simulink model "torque_version"  (R2022a)
settings: Solver=ode15s  StartTime=0.0  StopTime=5  MaxStep=1e-2  RelTol=1e-3
values from neighbouring files (symbols this model uses):
  Disturbance_F = -100    [controller_parameters.m]
  Disturbance_S = 100    [controller_parameters.m]
  k_gn = m*g/0.01    (= 41202)    [controller_parameters.m]
  k_gt = m*g/0.01    (= 41202)    [controller_parameters.m]
  Kd = 10    [controller_parameters.m]
  Kd_pitch = 8    [controller_parameters.m]
  Kp = 100    [controller_parameters.m]
  Kp_pitch = 100    [controller_parameters.m]
  m = 42    [controller_parameters.m]    (also in ground_reaction_params.m = 12)
  m_body = m_total/2    (= 20)    [controller_parameters.m]
  m_legs = m_total/2    (= 20)    [controller_parameters.m]
  mu_slide = 0.8    [controller_parameters.m]    (also in ground_reaction_params.m = 0.008)
  mu_stick = 0.9    [controller_parameters.m]    (also in ground_reaction_params.m = 0.009)
  v_gn_max = 0.03    [controller_parameters.m]
  v_gt_max = 0.03    [controller_parameters.m]
  vLimit = 0.01    [controller_parameters.m]    (also in ground_reaction_params.m = 0.001)
undefined symbols (not defined in the file or in its folder): Newton, Raphson, X, Y, Z
libraries: sm_lib x180, nesl_utility x113, simulink x32, simulink_extras x8
(part 3 of 8)

== system torque_version/Disturbance F ==
  Disturbance : Gain  Gain=Disturbance_F
  Step : Step  Time=2  SampleTime=0
  Step1 : Step  Time=2.1  After=-1  SampleTime=0
  Sum : Sum  Inputs=|++
  Disturbance Force [Frontal] : Outport
  wires:
  Step1/1 -> Sum/2
  Step/1 -> Sum/1
  Disturbance/1 -> Disturbance Force [Frontal]/1
  Sum/1 -> Disturbance/1

== system torque_version/Disturbance S ==
  Disturbance : Gain  Gain=Disturbance_S
  Step : Step  Time=2  SampleTime=0
  Step1 : Step  Time=2.1  After=-1  SampleTime=0
  Sum : Sum  Inputs=|++
  Disturbance Force [Sagittal] : Outport
  wires:
  Step1/1 -> Sum/2
  Step/1 -> Sum/1
  Disturbance/1 -> Disturbance Force [Sagittal]/1
  Sum/1 -> Disturbance/1

== system torque_version/Left Ankle Pitch PD Controller ==
  q : Inport
  dq : Inport  Port=2
  q_ref : Inport  Port=3
  dq_ref : Inport  Port=4
  Enable : EnablePort  StatesWhenEnabling=reset
  KD : Gain  Gain=Kd_pitch
  KP : Gain  Gain=Kp_pitch
  Saturation : Saturate  UpperLimit=40  LowerLimit=-40
  Sum : Sum  Inputs=|+-
  Sum1 : Sum  Inputs=+-|
  Sum2 : Sum  Inputs=|++
  Torque : Outport  OutputWhenDisabled=reset  InitialOutput=0
  wires:
  Saturation/1 -> Torque/1
  Sum2/1 -> Saturation/1
  q/1 -> Sum/2
  KP/1 -> Sum2/2
  dq/1 -> Sum1/2
  q_ref/1 -> Sum/1
  Sum1/1 -> KD/1
  dq_ref/1 -> Sum1/1
  Sum/1 -> KP/1
  KD/1 -> Sum2/1

== system torque_version/Left Ankle Roll PD Controller ==
  q : Inport
  dq : Inport  Port=2
  q_ref : Inport  Port=3
  dq_ref : Inport  Port=4
  Enable : EnablePort  StatesWhenEnabling=reset
  KD : Gain  Gain=Kd
  KP : Gain  Gain=Kp
  Saturation : Saturate  UpperLimit=20  LowerLimit=-20
  Sum : Sum  Inputs=|+-
  Sum1 : Sum  Inputs=+-|
  Sum2 : Sum  Inputs=|++
  Torque : Outport  OutputWhenDisabled=reset  InitialOutput=0
  wires:
  q/1 -> Sum/2
  KP/1 -> Sum2/2
  dq/1 -> Sum1/2
  q_ref/1 -> Sum/1
  Sum1/1 -> KD/1
  dq_ref/1 -> Sum1/1
  Sum/1 -> KP/1
  KD/1 -> Sum2/1
  Sum2/1 -> Saturation/1
  Saturation/1 -> Torque/1

== system torque_version/Left Hip Pitch PD Controller ==
  q : Inport
  dq : Inport  Port=2
  q_ref : Inport  Port=3
  dq_ref : Inport  Port=4
  Enable : EnablePort  StatesWhenEnabling=reset
  KD : Gain  Gain=Kd_pitch
  KP : Gain  Gain=Kp_pitch
  Saturation : Saturate  UpperLimit=50  LowerLimit=-50
  Sum : Sum  Inputs=|+-
  Sum1 : Sum  Inputs=+-|
  Sum2 : Sum  Inputs=|++
  Torque : Outport  OutputWhenDisabled=reset  InitialOutput=0
  wires:
  Saturation/1 -> Torque/1
  Sum2/1 -> Saturation/1
  q/1 -> Sum/2
  KP/1 -> Sum2/2
  dq/1 -> Sum1/2
  q_ref/1 -> Sum/1
  Sum1/1 -> KD/1
  dq_ref/1 -> Sum1/1
  Sum/1 -> KP/1
  KD/1 -> Sum2/1

== system torque_version/Left Hip Roll PD Controller ==
  q : Inport
  dq : Inport  Port=2
  q_ref : Inport  Port=3
  dq_ref : Inport  Port=4
  Enable : EnablePort  StatesWhenEnabling=reset
  KD : Gain  Gain=Kd
  KP : Gain  Gain=Kp
  Saturation : Saturate  UpperLimit=20  LowerLimit=-20
  Sum : Sum  Inputs=|+-
  Sum1 : Sum  Inputs=+-|
  Sum2 : Sum  Inputs=|++
  Torque : Outport  OutputWhenDisabled=reset  InitialOutput=0
  wires:
  KD/1 -> Sum2/1
  Sum/1 -> KP/1
  dq_ref/1 -> Sum1/1
  Sum1/1 -> KD/1
  q_ref/1 -> Sum/1
  dq/1 -> Sum1/2
  KP/1 -> Sum2/2
  q/1 -> Sum/2
  Sum2/1 -> Saturation/1
  Saturation/1 -> Torque/1

== system torque_version/Left Knee Pitch PD Controller ==
  q : Inport
  dq : Inport  Port=2
  q_ref : Inport  Port=3
  dq_ref : Inport  Port=4
  Enable : EnablePort  StatesWhenEnabling=reset
  KD : Gain  Gain=Kd_pitch
  KP : Gain  Gain=Kp_pitch
  Saturation : Saturate  UpperLimit=20  LowerLimit=-20
  Sum : Sum  Inputs=|+-
  Sum1 : Sum  Inputs=+-|
  Sum2 : Sum  Inputs=|++
  Torque : Outport  OutputWhenDisabled=reset  InitialOutput=0
  wires:
  KD/1 -> Sum2/1
  Sum/1 -> KP/1
  dq_ref/1 -> Sum1/1
  Sum1/1 -> KD/1
  q_ref/1 -> Sum/1
  dq/1 -> Sum1/2
  KP/1 -> Sum2/2
  q/1 -> Sum/2
  Sum2/1 -> Saturation/1
  Saturation/1 -> Torque/1

== system torque_version/Right Ankle Pitch PD Controller ==
  q : Inport
  dq : Inport  Port=2
  q_ref : Inport  Port=3
  dq_ref : Inport  Port=4
  Enable : EnablePort  StatesWhenEnabling=reset
  KD : Gain  Gain=Kd_pitch
  KP : Gain  Gain=Kp_pitch
  Saturation : Saturate  UpperLimit=40  LowerLimit=-40
  Sum : Sum  Inputs=|+-
  Sum1 : Sum  Inputs=+-|
  Sum2 : Sum  Inputs=|++
  Torque : Outport  OutputWhenDisabled=reset  InitialOutput=0
  wires:
  KD/1 -> Sum2/1
  Sum/1 -> KP/1
  dq_ref/1 -> Sum1/1
  Sum1/1 -> KD/1
  q_ref/1 -> Sum/1
  dq/1 -> Sum1/2
  KP/1 -> Sum2/2
  q/1 -> Sum/2
  Sum2/1 -> Saturation/1
  Saturation/1 -> Torque/1

== system torque_version/Right Ankle Roll PD Controller ==
  q : Inport
  dq : Inport  Port=2
  q_ref : Inport  Port=3
  dq_ref : Inport  Port=4
  Enable : EnablePort  StatesWhenEnabling=reset
  KD : Gain  Gain=Kd
  KP : Gain  Gain=Kp
  Saturation : Saturate  UpperLimit=20  LowerLimit=-20
  Sum : Sum  Inputs=|+-
  Sum1 : Sum  Inputs=+-|
  Sum2 : Sum  Inputs=|++
  Torque : Outport  OutputWhenDisabled=reset  InitialOutput=0
  wires:
  q/1 -> Sum/2
  KP/1 -> Sum2/2
  dq/1 -> Sum1/2
  q_ref/1 -> Sum/1
  Sum1/1 -> KD/1
  dq_ref/1 -> Sum1/1
  Sum/1 -> KP/1
  KD/1 -> Sum2/1
  Sum2/1 -> Saturation/1
  Saturation/1 -> Torque/1

== system torque_version/Right Hip Pitch PD Controller ==
  q : Inport
  dq : Inport  Port=2
  q_ref : Inport  Port=3
  dq_ref : Inport  Port=4
  Enable : EnablePort  StatesWhenEnabling=reset
  KD : Gain  Gain=Kd_pitch
  KP : Gain  Gain=Kp_pitch
  Saturation : Saturate  UpperLimit=50  LowerLimit=-50
  Sum : Sum  Inputs=|+-
  Sum1 : Sum  Inputs=+-|
  Sum2 : Sum  Inputs=|++
  Torque : Outport  OutputWhenDisabled=reset  InitialOutput=0
  wires:
  KD/1 -> Sum2/1
  Sum/1 -> KP/1
  dq_ref/1 -> Sum1/1
  Sum1/1 -> KD/1
  q_ref/1 -> Sum/1
  dq/1 -> Sum1/2
  KP/1 -> Sum2/2
  q/1 -> Sum/2
  Sum2/1 -> Saturation/1
  Saturation/1 -> Torque/1

== system torque_version/Right Hip Roll PD Controller ==
  q : Inport
  dq : Inport  Port=2
  q_ref : Inport  Port=3
  dq_ref : Inport  Port=4
  Enable : EnablePort  StatesWhenEnabling=reset
  KD : Gain  Gain=Kd
  KP : Gain  Gain=Kp
  Saturation : Saturate  UpperLimit=20  LowerLimit=-20
  Sum : Sum  Inputs=|+-
  Sum1 : Sum  Inputs=+-|
  Sum2 : Sum  Inputs=|++
  Torque : Outport  OutputWhenDisabled=reset  InitialOutput=0
  wires:
  q/1 -> Sum/2
  KP/1 -> Sum2/2
  dq/1 -> Sum1/2
  q_ref/1 -> Sum/1
  Sum1/1 -> KD/1
  dq_ref/1 -> Sum1/1
  Sum/1 -> KP/1
  KD/1 -> Sum2/1
  Sum2/1 -> Saturation/1
  Saturation/1 -> Torque/1

== system torque_version/Right Knee Pitch PD Controller ==
  q : Inport
  dq : Inport  Port=2
  q_ref : Inport  Port=3
  dq_ref : Inport  Port=4
  Enable : EnablePort  StatesWhenEnabling=reset
  KD : Gain  Gain=Kd_pitch
  KP : Gain  Gain=Kp_pitch
  Saturation : Saturate  UpperLimit=20  LowerLimit=-20
  Sum : Sum  Inputs=|+-
  Sum1 : Sum  Inputs=+-|
  Sum2 : Sum  Inputs=|++
  Torque : Outport  OutputWhenDisabled=reset  InitialOutput=0
  wires:
  Saturation/1 -> Torque/1
  Sum2/1 -> Saturation/1
  q/1 -> Sum/2
  KP/1 -> Sum2/2
  dq/1 -> Sum1/2
  q_ref/1 -> Sum/1
  Sum1/1 -> KD/1
  dq_ref/1 -> Sum1/1
  Sum/1 -> KP/1
  KD/1 -> Sum2/1

== system torque_version/Bipedal Model with Torque Control/Left Ball C1 ==
  note: 3D Ground Interaction Model
  Ground : Inport
  3D Contact : Subsystem
  Constant1 : Constant  Value=[0 0 1]
  Demux : Demux  Outputs=3
  Demux1 : Demux  Outputs=3
  External Force and Torque : sm_lib/Forces and Torques/External Force and Torque  ForceResolutionFrame=World  EnableForceX=on  EnableForceY=on  EnableForceZ=on  EnableForce=off  TorqueResolutionFrame=AttachedFrame  EnableTorqueX=off  EnableTorqueY=off  EnableTorqueZ=off  EnableTorque=off
  Mux : Mux  Inputs=3
  Mux1 : Mux  Inputs=3
  Mux2 : Mux  Inputs=3
  PS-Simulink Converter : nesl_utility/PS-Simulink Converter  PhysicalDomain=network_engine_domain  SubClassName=ps_output  LeftPortType=input  RightPortType=output  PseudoPeriodic=off  Frequencies=[]  VectorFormat=1-D array  Unit=m  AffineConversion=off
      settings: SourceProductBaseCode=PW,SS
  PS-Simulink Converter1 : nesl_utility/PS-Simulink Converter  PhysicalDomain=network_engine_domain  SubClassName=ps_output  LeftPortType=input  RightPortType=output  PseudoPeriodic=off  Frequencies=[]  VectorFormat=1-D array  Unit=m  AffineConversion=off
      settings: SourceProductBaseCode=PW,SS
  PS-Simulink Converter2 : nesl_utility/PS-Simulink Converter  PhysicalDomain=network_engine_domain  SubClassName=ps_output  LeftPortType=input  RightPortType=output  PseudoPeriodic=off  Frequencies=[]  VectorFormat=1-D array  Unit=m  AffineConversion=off
      settings: SourceProductBaseCode=PW,SS
  PS-Simulink Converter3 : nesl_utility/PS-Simulink Converter  PhysicalDomain=network_engine_domain  SubClassName=ps_output  LeftPortType=input  RightPortType=output  PseudoPeriodic=off  Frequencies=[]  VectorFormat=1-D array  Unit=m/s  AffineConversion=off
      settings: SourceProductBaseCode=PW,SS
  PS-Simulink Converter4 : nesl_utility/PS-Simulink Converter  PhysicalDomain=network_engine_domain  SubClassName=ps_output  LeftPortType=input  RightPortType=output  PseudoPeriodic=off  Frequencies=[]  VectorFormat=1-D array  Unit=m/s  AffineConversion=off
      settings: SourceProductBaseCode=PW,SS
  PS-Simulink Converter5 : nesl_utility/PS-Simulink Converter  PhysicalDomain=network_engine_domain  SubClassName=ps_output  LeftPortType=input  RightPortType=output  PseudoPeriodic=off  Frequencies=[]  VectorFormat=1-D array  Unit=m/s  AffineConversion=off
      settings: SourceProductBaseCode=PW,SS
  Simulink-PS Converter : nesl_utility/Simulink-PS Converter  PhysicalDomain=network_engine_domain  SubClassName=ps_input  LeftPortType=input  RightPortType=output  PseudoPeriodic=off  Frequencies=[]  NoiseDistribution=none  NoiseParameters=[]  Unit=N  AffineConversion=off  FilteringAndDerivatives=provide  SimscapeFilterOrder=1  InputFilterTimeConstant=0.001  UdotUserProvided=0
      settings: SourceProductBaseCode=PW,SS
  Simulink-PS Converter1 : nesl_utility/Simulink-PS Converter  PhysicalDomain=network_engine_domain  SubClassName=ps_input  LeftPortType=input  RightPortType=output  PseudoPeriodic=off  Frequencies=[]  NoiseDistribution=none  NoiseParameters=[]  Unit=N  AffineConversion=off  FilteringAndDerivatives=provide  SimscapeFilterOrder=1  InputFilterTimeConstant=0.001  UdotUserProvided=0
      settings: SourceProductBaseCode=PW,SS
  Simulink-PS Converter2 : nesl_utility/Simulink-PS Converter  PhysicalDomain=network_engine_domain  SubClassName=ps_input  LeftPortType=input  RightPortType=output  PseudoPeriodic=off  Frequencies=[]  NoiseDistribution=none  NoiseParameters=[]  Unit=N  AffineConversion=off  FilteringAndDerivatives=provide  SimscapeFilterOrder=1  InputFilterTimeConstant=0.001  UdotUserProvided=0
      settings: SourceProductBaseCode=PW,SS
  Sum : Sum  Inputs=|+-
  Sum1 : Sum
  Terminator : Terminator
  Transform Sensor : sm_lib/Frames and Transforms/Transform Sensor  MeasurementFrame=World  SenseAngle=off  SenseAxis=off  SenseAngle1=off  SenseAngle2=off  SenseAngle3=off  SenseQ=off  SenseR=off  SenseOmegaX=off  SenseOmegaY=off  SenseOmegaZ=off  SenseOmega1=off  SenseOmega2=off  SenseOmega3=off  SenseQDot=off  SenseRDot=off  SenseAlphaX=off  SenseAlphaY=off  SenseAlphaZ=off  SenseAlpha1=off  SenseAlpha2=off  SenseAlpha3=off  SenseQDDot=off  SenseRDDot=off  SenseX=on  SenseY=on  SenseZ=on  SenseRad=off  SenseAzim=off  SenseDist=off  SenseInc=off  SenseXDot=on  SenseYDot=on  SenseZDot=on  SenseRadDot=off  SenseAzimDot=off  SenseDistDot=off  SenseIncDot=off  SenseXDDot=off  SenseYDDot=off  SenseZDDot=off  SenseRadDDot=off  SenseAzimDDot=off  SenseDistDDot=off  SenseIncDDot=off
  contact? : simulink/Logic and Bit Operations/Compare To Zero  relop=<=  OutDataTypeStr=boolean
  z : Selector  InputPortWidth=3  IndexOptions=Index vector (dialog)  Indices=3  OutputSizes=1
  F : PMIOPort  Side=Left
  WorldFrame : PMIOPort  Port=2  Side=Left
  RBallCnt : Outport
  GRF [N N N] : Outport  Port=2
  GRFt [N N N] : Outport  Port=3
  GRFn [N N N] : Outport  Port=4
  wires:
  contact?/1 -> 3D Contact/Enable, RBallCnt/1  "cnt"
  Mux2/1 -> 3D Contact/4(vVec [m/s m/s m/s])
  3D Contact/1(FnVec [N N N]) -> Sum1/1, GRFn [N N N]/1
  3D Contact/2(FtVec [N N N]) -> Sum1/2, GRFt [N N N]/1
  Sum1/1 -> GRF [N N N]/1, Demux1/1
  Sum/1 -> contact?/1
  z/1 -> Sum/1
  Ground/1 -> Mux/3, Sum/2  "EnvHeight"
  Constant1/1 -> 3D Contact/2(nVec [m m m])  "Normal Vector nVec"
  Mux1/1 -> 3D Contact/3(pVec [m m m]), z/1, Demux/1  "Reference Point RefPt"
  Demux/1 -> Mux/1
  Mux/1 -> 3D Contact/1(RefPt [m m m])
  Demux1/1 -> Simulink-PS Converter/1
  Demux1/2 -> Simulink-PS Converter1/1
  Demux1/3 -> Simulink-PS Converter2/1
  PS-Simulink Converter1/1 -> Mux1/2
  PS-Simulink Converter/1 -> Mux1/1
  PS-Simulink Converter2/1 -> Mux1/3
  PS-Simulink Converter3/1 -> Mux2/1
  PS-Simulink Converter4/1 -> Mux2/2
  PS-Simulink Converter5/1 -> Mux2/3
  Demux/3 -> Terminator/1
  Demux/2 -> Mux/2
  connections:
  Transform Sensor/RConn1 -- External Force and Torque/RConn1 -- F/RConn1
  Simulink-PS Converter/RConn1 -- External Force and Torque/LConn1
  Simulink-PS Converter1/RConn1 -- External Force and Torque/LConn2
  Simulink-PS Converter2/RConn1 -- External Force and Torque/LConn3
  WorldFrame/RConn1 -- Transform Sensor/LConn1
  PS-Simulink Converter/LConn1 -- Transform Sensor/RConn2
  PS-Simulink Converter1/LConn1 -- Transform Sensor/RConn3
  PS-Simulink Converter2/LConn1 -- Transform Sensor/RConn4
  PS-Simulink Converter3/LConn1 -- Transform Sensor/RConn5
  PS-Simulink Converter4/LConn1 -- Transform Sensor/RConn6
  PS-Simulink Converter5/LConn1 -- Transform Sensor/RConn7

== system torque_version/Bipedal Model with Torque Control/Left Ball C2 ==
  note: 3D Ground Interaction Model
  Ground : Inport
  3D Contact : Subsystem
  Constant1 : Constant  Value=[0 0 1]
  Demux : Demux  Outputs=3
  Demux1 : Demux  Outputs=3
  External Force and Torque : sm_lib/Forces and Torques/External Force and Torque  ForceResolutionFrame=World  EnableForceX=on  EnableForceY=on  EnableForceZ=on  EnableForce=off  TorqueResolutionFrame=AttachedFrame  EnableTorqueX=off  EnableTorqueY=off  EnableTorqueZ=off  EnableTorque=off
  Mux : Mux  Inputs=3
  Mux1 : Mux  Inputs=3
  Mux2 : Mux  Inputs=3
  PS-Simulink Converter : nesl_utility/PS-Simulink Converter  PhysicalDomain=network_engine_domain  SubClassName=ps_output  LeftPortType=input  RightPortType=output  PseudoPeriodic=off  Frequencies=[]  VectorFormat=1-D array  Unit=m  AffineConversion=off
      settings: SourceProductBaseCode=PW,SS
  PS-Simulink Converter1 : nesl_utility/PS-Simulink Converter  PhysicalDomain=network_engine_domain  SubClassName=ps_output  LeftPortType=input  RightPortType=output  PseudoPeriodic=off  Frequencies=[]  VectorFormat=1-D array  Unit=m  AffineConversion=off
      settings: SourceProductBaseCode=PW,SS
  PS-Simulink Converter2 : nesl_utility/PS-Simulink Converter  PhysicalDomain=network_engine_domain  SubClassName=ps_output  LeftPortType=input  RightPortType=output  PseudoPeriodic=off  Frequencies=[]  VectorFormat=1-D array  Unit=m  AffineConversion=off
      settings: SourceProductBaseCode=PW,SS
  PS-Simulink Converter3 : nesl_utility/PS-Simulink Converter  PhysicalDomain=network_engine_domain  SubClassName=ps_output  LeftPortType=input  RightPortType=output  PseudoPeriodic=off  Frequencies=[]  VectorFormat=1-D array  Unit=m/s  AffineConversion=off
      settings: SourceProductBaseCode=PW,SS
  PS-Simulink Converter4 : nesl_utility/PS-Simulink Converter  PhysicalDomain=network_engine_domain  SubClassName=ps_output  LeftPortType=input  RightPortType=output  PseudoPeriodic=off  Frequencies=[]  VectorFormat=1-D array  Unit=m/s  AffineConversion=off
      settings: SourceProductBaseCode=PW,SS
  PS-Simulink Converter5 : nesl_utility/PS-Simulink Converter  PhysicalDomain=network_engine_domain  SubClassName=ps_output  LeftPortType=input  RightPortType=output  PseudoPeriodic=off  Frequencies=[]  VectorFormat=1-D array  Unit=m/s  AffineConversion=off
      settings: SourceProductBaseCode=PW,SS
  Simulink-PS Converter : nesl_utility/Simulink-PS Converter  PhysicalDomain=network_engine_domain  SubClassName=ps_input  LeftPortType=input  RightPortType=output  PseudoPeriodic=off  Frequencies=[]  NoiseDistribution=none  NoiseParameters=[]  Unit=N  AffineConversion=off  FilteringAndDerivatives=provide  SimscapeFilterOrder=1  InputFilterTimeConstant=0.001  UdotUserProvided=0
      settings: SourceProductBaseCode=PW,SS
  Simulink-PS Converter1 : nesl_utility/Simulink-PS Converter  PhysicalDomain=network_engine_domain  SubClassName=ps_input  LeftPortType=input  RightPortType=output  PseudoPeriodic=off  Frequencies=[]  NoiseDistribution=none  NoiseParameters=[]  Unit=N  AffineConversion=off  FilteringAndDerivatives=provide  SimscapeFilterOrder=1  InputFilterTimeConstant=0.001  UdotUserProvided=0
      settings: SourceProductBaseCode=PW,SS
  Simulink-PS Converter2 : nesl_utility/Simulink-PS Converter  PhysicalDomain=network_engine_domain  SubClassName=ps_input  LeftPortType=input  RightPortType=output  PseudoPeriodic=off  Frequencies=[]  NoiseDistribution=none  NoiseParameters=[]  Unit=N  AffineConversion=off  FilteringAndDerivatives=provide  SimscapeFilterOrder=1  InputFilterTimeConstant=0.001  UdotUserProvided=0
      settings: SourceProductBaseCode=PW,SS
  Sum : Sum  Inputs=|+-
  Sum1 : Sum
  Terminator : Terminator
  Transform Sensor : sm_lib/Frames and Transforms/Transform Sensor  MeasurementFrame=World  SenseAngle=off  SenseAxis=off  SenseAngle1=off  SenseAngle2=off  SenseAngle3=off  SenseQ=off  SenseR=off  SenseOmegaX=off  SenseOmegaY=off  SenseOmegaZ=off  SenseOmega1=off  SenseOmega2=off  SenseOmega3=off  SenseQDot=off  SenseRDot=off  SenseAlphaX=off  SenseAlphaY=off  SenseAlphaZ=off  SenseAlpha1=off  SenseAlpha2=off  SenseAlpha3=off  SenseQDDot=off  SenseRDDot=off  SenseX=on  SenseY=on  SenseZ=on  SenseRad=off  SenseAzim=off  SenseDist=off  SenseInc=off  SenseXDot=on  SenseYDot=on  SenseZDot=on  SenseRadDot=off  SenseAzimDot=off  SenseDistDot=off  SenseIncDot=off  SenseXDDot=off  SenseYDDot=off  SenseZDDot=off  SenseRadDDot=off  SenseAzimDDot=off  SenseDistDDot=off  SenseIncDDot=off
  contact? : simulink/Logic and Bit Operations/Compare To Zero  relop=<=  OutDataTypeStr=boolean
  z : Selector  InputPortWidth=3  IndexOptions=Index vector (dialog)  Indices=3  OutputSizes=1
  F : PMIOPort  Side=Left
  WorldFrame : PMIOPort  Port=2  Side=Left
  RBallCnt : Outport
  GRF [N N N] : Outport  Port=2
  GRFt [N N N] : Outport  Port=3
  GRFn [N N N] : Outport  Port=4
  wires:
  Demux/2 -> Mux/2
  Demux/3 -> Terminator/1
  PS-Simulink Converter5/1 -> Mux2/3
  PS-Simulink Converter4/1 -> Mux2/2
  PS-Simulink Converter3/1 -> Mux2/1
  PS-Simulink Converter2/1 -> Mux1/3
  PS-Simulink Converter/1 -> Mux1/1
  PS-Simulink Converter1/1 -> Mux1/2
  Demux1/3 -> Simulink-PS Converter2/1
  Demux1/2 -> Simulink-PS Converter1/1
  Demux1/1 -> Simulink-PS Converter/1
  Mux/1 -> 3D Contact/1(RefPt [m m m])
  Demux/1 -> Mux/1
  Mux1/1 -> Demux/1, z/1, 3D Contact/3(pVec [m m m])  "Reference Point RefPt"
  Constant1/1 -> 3D Contact/2(nVec [m m m])  "Normal Vector nVec"
  Ground/1 -> Sum/2, Mux/3  "EnvHeight"
  z/1 -> Sum/1
  Sum/1 -> contact?/1
  Sum1/1 -> Demux1/1, GRF [N N N]/1
  3D Contact/2(FtVec [N N N]) -> GRFt [N N N]/1, Sum1/2
  3D Contact/1(FnVec [N N N]) -> GRFn [N N N]/1, Sum1/1
  Mux2/1 -> 3D Contact/4(vVec [m/s m/s m/s])
  contact?/1 -> RBallCnt/1, 3D Contact/Enable  "cnt"
  connections:
  PS-Simulink Converter5/LConn1 -- Transform Sensor/RConn7
  PS-Simulink Converter4/LConn1 -- Transform Sensor/RConn6
  PS-Simulink Converter3/LConn1 -- Transform Sensor/RConn5
  PS-Simulink Converter2/LConn1 -- Transform Sensor/RConn4
  PS-Simulink Converter1/LConn1 -- Transform Sensor/RConn3
  PS-Simulink Converter/LConn1 -- Transform Sensor/RConn2
  WorldFrame/RConn1 -- Transform Sensor/LConn1
  Simulink-PS Converter2/RConn1 -- External Force and Torque/LConn3
  Simulink-PS Converter1/RConn1 -- External Force and Torque/LConn2
  Simulink-PS Converter/RConn1 -- External Force and Torque/LConn1
  F/RConn1 -- External Force and Torque/RConn1 -- Transform Sensor/RConn1

== system torque_version/Bipedal Model with Torque Control/Left Ball C3 ==
  note: 3D Ground Interaction Model
  Ground : Inport
  3D Contact : Subsystem
  Constant1 : Constant  Value=[0 0 1]
  Demux : Demux  Outputs=3
  Demux1 : Demux  Outputs=3
  External Force and Torque : sm_lib/Forces and Torques/External Force and Torque  ForceResolutionFrame=World  EnableForceX=on  EnableForceY=on  EnableForceZ=on  EnableForce=off  TorqueResolutionFrame=AttachedFrame  EnableTorqueX=off  EnableTorqueY=off  EnableTorqueZ=off  EnableTorque=off
  Mux : Mux  Inputs=3
  Mux1 : Mux  Inputs=3
  Mux2 : Mux  Inputs=3
  PS-Simulink Converter : nesl_utility/PS-Simulink Converter  PhysicalDomain=network_engine_domain  SubClassName=ps_output  LeftPortType=input  RightPortType=output  PseudoPeriodic=off  Frequencies=[]  VectorFormat=1-D array  Unit=m  AffineConversion=off
      settings: SourceProductBaseCode=PW,SS
  PS-Simulink Converter1 : nesl_utility/PS-Simulink Converter  PhysicalDomain=network_engine_domain  SubClassName=ps_output  LeftPortType=input  RightPortType=output  PseudoPeriodic=off  Frequencies=[]  VectorFormat=1-D array  Unit=m  AffineConversion=off
      settings: SourceProductBaseCode=PW,SS
  PS-Simulink Converter2 : nesl_utility/PS-Simulink Converter  PhysicalDomain=network_engine_domain  SubClassName=ps_output  LeftPortType=input  RightPortType=output  PseudoPeriodic=off  Frequencies=[]  VectorFormat=1-D array  Unit=m  AffineConversion=off
      settings: SourceProductBaseCode=PW,SS
  PS-Simulink Converter3 : nesl_utility/PS-Simulink Converter  PhysicalDomain=network_engine_domain  SubClassName=ps_output  LeftPortType=input  RightPortType=output  PseudoPeriodic=off  Frequencies=[]  VectorFormat=1-D array  Unit=m/s  AffineConversion=off
      settings: SourceProductBaseCode=PW,SS
  PS-Simulink Converter4 : nesl_utility/PS-Simulink Converter  PhysicalDomain=network_engine_domain  SubClassName=ps_output  LeftPortType=input  RightPortType=output  PseudoPeriodic=off  Frequencies=[]  VectorFormat=1-D array  Unit=m/s  AffineConversion=off
      settings: SourceProductBaseCode=PW,SS
  PS-Simulink Converter5 : nesl_utility/PS-Simulink Converter  PhysicalDomain=network_engine_domain  SubClassName=ps_output  LeftPortType=input  RightPortType=output  PseudoPeriodic=off  Frequencies=[]  VectorFormat=1-D array  Unit=m/s  AffineConversion=off
      settings: SourceProductBaseCode=PW,SS
  Simulink-PS Converter : nesl_utility/Simulink-PS Converter  PhysicalDomain=network_engine_domain  SubClassName=ps_input  LeftPortType=input  RightPortType=output  PseudoPeriodic=off  Frequencies=[]  NoiseDistribution=none  NoiseParameters=[]  Unit=N  AffineConversion=off  FilteringAndDerivatives=provide  SimscapeFilterOrder=1  InputFilterTimeConstant=0.001  UdotUserProvided=0
      settings: SourceProductBaseCode=PW,SS
  Simulink-PS Converter1 : nesl_utility/Simulink-PS Converter  PhysicalDomain=network_engine_domain  SubClassName=ps_input  LeftPortType=input  RightPortType=output  PseudoPeriodic=off  Frequencies=[]  NoiseDistribution=none  NoiseParameters=[]  Unit=N  AffineConversion=off  FilteringAndDerivatives=provide  SimscapeFilterOrder=1  InputFilterTimeConstant=0.001  UdotUserProvided=0
      settings: SourceProductBaseCode=PW,SS
  Simulink-PS Converter2 : nesl_utility/Simulink-PS Converter  PhysicalDomain=network_engine_domain  SubClassName=ps_input  LeftPortType=input  RightPortType=output  PseudoPeriodic=off  Frequencies=[]  NoiseDistribution=none  NoiseParameters=[]  Unit=N  AffineConversion=off  FilteringAndDerivatives=provide  SimscapeFilterOrder=1  InputFilterTimeConstant=0.001  UdotUserProvided=0
      settings: SourceProductBaseCode=PW,SS
  Sum : Sum  Inputs=|+-
  Sum1 : Sum
  Terminator : Terminator
  Transform Sensor : sm_lib/Frames and Transforms/Transform Sensor  MeasurementFrame=World  SenseAngle=off  SenseAxis=off  SenseAngle1=off  SenseAngle2=off  SenseAngle3=off  SenseQ=off  SenseR=off  SenseOmegaX=off  SenseOmegaY=off  SenseOmegaZ=off  SenseOmega1=off  SenseOmega2=off  SenseOmega3=off  SenseQDot=off  SenseRDot=off  SenseAlphaX=off  SenseAlphaY=off  SenseAlphaZ=off  SenseAlpha1=off  SenseAlpha2=off  SenseAlpha3=off  SenseQDDot=off  SenseRDDot=off  SenseX=on  SenseY=on  SenseZ=on  SenseRad=off  SenseAzim=off  SenseDist=off  SenseInc=off  SenseXDot=on  SenseYDot=on  SenseZDot=on  SenseRadDot=off  SenseAzimDot=off  SenseDistDot=off  SenseIncDot=off  SenseXDDot=off  SenseYDDot=off  SenseZDDot=off  SenseRadDDot=off  SenseAzimDDot=off  SenseDistDDot=off  SenseIncDDot=off
  contact? : simulink/Logic and Bit Operations/Compare To Zero  relop=<=  OutDataTypeStr=boolean
  z : Selector  InputPortWidth=3  IndexOptions=Index vector (dialog)  Indices=3  OutputSizes=1
  F : PMIOPort  Side=Left
  WorldFrame : PMIOPort  Port=2  Side=Left
  RBallCnt : Outport
  GRF [N N N] : Outport  Port=2
  GRFt [N N N] : Outport  Port=3
  GRFn [N N N] : Outport  Port=4
  wires:
  contact?/1 -> 3D Contact/Enable, RBallCnt/1  "cnt"
  Mux2/1 -> 3D Contact/4(vVec [m/s m/s m/s])
  3D Contact/1(FnVec [N N N]) -> Sum1/1, GRFn [N N N]/1
  3D Contact/2(FtVec [N N N]) -> Sum1/2, GRFt [N N N]/1
  Sum1/1 -> GRF [N N N]/1, Demux1/1
  Sum/1 -> contact?/1
  z/1 -> Sum/1
  Ground/1 -> Mux/3, Sum/2  "EnvHeight"
  Constant1/1 -> 3D Contact/2(nVec [m m m])  "Normal Vector nVec"
  Mux1/1 -> 3D Contact/3(pVec [m m m]), z/1, Demux/1  "Reference Point RefPt"
  Demux/1 -> Mux/1
  Mux/1 -> 3D Contact/1(RefPt [m m m])
  Demux1/1 -> Simulink-PS Converter/1
  Demux1/2 -> Simulink-PS Converter1/1
  Demux1/3 -> Simulink-PS Converter2/1
  PS-Simulink Converter1/1 -> Mux1/2
  PS-Simulink Converter/1 -> Mux1/1
  PS-Simulink Converter2/1 -> Mux1/3
  PS-Simulink Converter3/1 -> Mux2/1
  PS-Simulink Converter4/1 -> Mux2/2
  PS-Simulink Converter5/1 -> Mux2/3
  Demux/3 -> Terminator/1
  Demux/2 -> Mux/2
  connections:
  Transform Sensor/RConn1 -- External Force and Torque/RConn1 -- F/RConn1
  Simulink-PS Converter/RConn1 -- External Force and Torque/LConn1
  Simulink-PS Converter1/RConn1 -- External Force and Torque/LConn2
  Simulink-PS Converter2/RConn1 -- External Force and Torque/LConn3
  WorldFrame/RConn1 -- Transform Sensor/LConn1
  PS-Simulink Converter/LConn1 -- Transform Sensor/RConn2
  PS-Simulink Converter1/LConn1 -- Transform Sensor/RConn3
  PS-Simulink Converter2/LConn1 -- Transform Sensor/RConn4
  PS-Simulink Converter3/LConn1 -- Transform Sensor/RConn5
  PS-Simulink Converter4/LConn1 -- Transform Sensor/RConn6
  PS-Simulink Converter5/LConn1 -- Transform Sensor/RConn7

== system torque_version/Bipedal Model with Torque Control/Left Ball C4 ==
  note: 3D Ground Interaction Model
  Ground : Inport
  3D Contact : Subsystem
  Constant1 : Constant  Value=[0 0 1]
  Demux : Demux  Outputs=3
  Demux1 : Demux  Outputs=3
  External Force and Torque : sm_lib/Forces and Torques/External Force and Torque  ForceResolutionFrame=World  EnableForceX=on  EnableForceY=on  EnableForceZ=on  EnableForce=off  TorqueResolutionFrame=AttachedFrame  EnableTorqueX=off  EnableTorqueY=off  EnableTorqueZ=off  EnableTorque=off
  Mux : Mux  Inputs=3
  Mux1 : Mux  Inputs=3
  Mux2 : Mux  Inputs=3
  PS-Simulink Converter : nesl_utility/PS-Simulink Converter  PhysicalDomain=network_engine_domain  SubClassName=ps_output  LeftPortType=input  RightPortType=output  PseudoPeriodic=off  Frequencies=[]  VectorFormat=1-D array  Unit=m  AffineConversion=off
      settings: SourceProductBaseCode=PW,SS
  PS-Simulink Converter1 : nesl_utility/PS-Simulink Converter  PhysicalDomain=network_engine_domain  SubClassName=ps_output  LeftPortType=input  RightPortType=output  PseudoPeriodic=off  Frequencies=[]  VectorFormat=1-D array  Unit=m  AffineConversion=off
      settings: SourceProductBaseCode=PW,SS
  PS-Simulink Converter2 : nesl_utility/PS-Simulink Converter  PhysicalDomain=network_engine_domain  SubClassName=ps_output  LeftPortType=input  RightPortType=output  PseudoPeriodic=off  Frequencies=[]  VectorFormat=1-D array  Unit=m  AffineConversion=off
      settings: SourceProductBaseCode=PW,SS
  PS-Simulink Converter3 : nesl_utility/PS-Simulink Converter  PhysicalDomain=network_engine_domain  SubClassName=ps_output  LeftPortType=input  RightPortType=output  PseudoPeriodic=off  Frequencies=[]  VectorFormat=1-D array  Unit=m/s  AffineConversion=off
      settings: SourceProductBaseCode=PW,SS
  PS-Simulink Converter4 : nesl_utility/PS-Simulink Converter  PhysicalDomain=network_engine_domain  SubClassName=ps_output  LeftPortType=input  RightPortType=output  PseudoPeriodic=off  Frequencies=[]  VectorFormat=1-D array  Unit=m/s  AffineConversion=off
      settings: SourceProductBaseCode=PW,SS
  PS-Simulink Converter5 : nesl_utility/PS-Simulink Converter  PhysicalDomain=network_engine_domain  SubClassName=ps_output  LeftPortType=input  RightPortType=output  PseudoPeriodic=off  Frequencies=[]  VectorFormat=1-D array  Unit=m/s  AffineConversion=off
      settings: SourceProductBaseCode=PW,SS
  Simulink-PS Converter : nesl_utility/Simulink-PS Converter  PhysicalDomain=network_engine_domain  SubClassName=ps_input  LeftPortType=input  RightPortType=output  PseudoPeriodic=off  Frequencies=[]  NoiseDistribution=none  NoiseParameters=[]  Unit=N  AffineConversion=off  FilteringAndDerivatives=provide  SimscapeFilterOrder=1  InputFilterTimeConstant=0.001  UdotUserProvided=0
      settings: SourceProductBaseCode=PW,SS
  Simulink-PS Converter1 : nesl_utility/Simulink-PS Converter  PhysicalDomain=network_engine_domain  SubClassName=ps_input  LeftPortType=input  RightPortType=output  PseudoPeriodic=off  Frequencies=[]  NoiseDistribution=none  NoiseParameters=[]  Unit=N  AffineConversion=off  FilteringAndDerivatives=provide  SimscapeFilterOrder=1  InputFilterTimeConstant=0.001  UdotUserProvided=0
      settings: SourceProductBaseCode=PW,SS
  Simulink-PS Converter2 : nesl_utility/Simulink-PS Converter  PhysicalDomain=network_engine_domain  SubClassName=ps_input  LeftPortType=input  RightPortType=output  PseudoPeriodic=off  Frequencies=[]  NoiseDistribution=none  NoiseParameters=[]  Unit=N  AffineConversion=off  FilteringAndDerivatives=provide  SimscapeFilterOrder=1  InputFilterTimeConstant=0.001  UdotUserProvided=0
      settings: SourceProductBaseCode=PW,SS
  Sum : Sum  Inputs=|+-
  Sum1 : Sum
  Terminator : Terminator
  Transform Sensor : sm_lib/Frames and Transforms/Transform Sensor  MeasurementFrame=World  SenseAngle=off  SenseAxis=off  SenseAngle1=off  SenseAngle2=off  SenseAngle3=off  SenseQ=off  SenseR=off  SenseOmegaX=off  SenseOmegaY=off  SenseOmegaZ=off  SenseOmega1=off  SenseOmega2=off  SenseOmega3=off  SenseQDot=off  SenseRDot=off  SenseAlphaX=off  SenseAlphaY=off  SenseAlphaZ=off  SenseAlpha1=off  SenseAlpha2=off  SenseAlpha3=off  SenseQDDot=off  SenseRDDot=off  SenseX=on  SenseY=on  SenseZ=on  SenseRad=off  SenseAzim=off  SenseDist=off  SenseInc=off  SenseXDot=on  SenseYDot=on  SenseZDot=on  SenseRadDot=off  SenseAzimDot=off  SenseDistDot=off  SenseIncDot=off  SenseXDDot=off  SenseYDDot=off  SenseZDDot=off  SenseRadDDot=off  SenseAzimDDot=off  SenseDistDDot=off  SenseIncDDot=off
  contact? : simulink/Logic and Bit Operations/Compare To Zero  relop=<=  OutDataTypeStr=boolean
  z : Selector  InputPortWidth=3  IndexOptions=Index vector (dialog)  Indices=3  OutputSizes=1
  F : PMIOPort  Side=Left
  WorldFrame : PMIOPort  Port=2  Side=Left
  RBallCnt : Outport
  GRF [N N N] : Outport  Port=2
  GRFt [N N N] : Outport  Port=3
  GRFn [N N N] : Outport  Port=4
  wires:
  Demux/2 -> Mux/2
  Demux/3 -> Terminator/1
  PS-Simulink Converter5/1 -> Mux2/3
  PS-Simulink Converter4/1 -> Mux2/2
  PS-Simulink Converter3/1 -> Mux2/1
  PS-Simulink Converter2/1 -> Mux1/3
  PS-Simulink Converter/1 -> Mux1/1
  PS-Simulink Converter1/1 -> Mux1/2
  Demux1/3 -> Simulink-PS Converter2/1
  Demux1/2 -> Simulink-PS Converter1/1
  Demux1/1 -> Simulink-PS Converter/1
  Mux/1 -> 3D Contact/1(RefPt [m m m])
  Demux/1 -> Mux/1
  Mux1/1 -> Demux/1, z/1, 3D Contact/3(pVec [m m m])  "Reference Point RefPt"
  Constant1/1 -> 3D Contact/2(nVec [m m m])  "Normal Vector nVec"
  Ground/1 -> Sum/2, Mux/3  "EnvHeight"
  z/1 -> Sum/1
  Sum/1 -> contact?/1
  Sum1/1 -> Demux1/1, GRF [N N N]/1
  3D Contact/2(FtVec [N N N]) -> GRFt [N N N]/1, Sum1/2
  3D Contact/1(FnVec [N N N]) -> GRFn [N N N]/1, Sum1/1
  Mux2/1 -> 3D Contact/4(vVec [m/s m/s m/s])
  contact?/1 -> RBallCnt/1, 3D Contact/Enable  "cnt"
  connections:
  PS-Simulink Converter5/LConn1 -- Transform Sensor/RConn7
  PS-Simulink Converter4/LConn1 -- Transform Sensor/RConn6
  PS-Simulink Converter3/LConn1 -- Transform Sensor/RConn5
  PS-Simulink Converter2/LConn1 -- Transform Sensor/RConn4
  PS-Simulink Converter1/LConn1 -- Transform Sensor/RConn3
  PS-Simulink Converter/LConn1 -- Transform Sensor/RConn2
  WorldFrame/RConn1 -- Transform Sensor/LConn1
  Simulink-PS Converter2/RConn1 -- External Force and Torque/LConn3
  Simulink-PS Converter1/RConn1 -- External Force and Torque/LConn2
  Simulink-PS Converter/RConn1 -- External Force and Torque/LConn1
  F/RConn1 -- External Force and Torque/RConn1 -- Transform Sensor/RConn1

== system torque_version/Bipedal Model with Torque Control/Right Ball C1 ==
  note: 3D Ground Interaction Model
  Ground : Inport
  3D Contact : Subsystem
  Constant1 : Constant  Value=[0 0 1]
  Demux : Demux  Outputs=3
  Demux1 : Demux  Outputs=3
  External Force and Torque : sm_lib/Forces and Torques/External Force and Torque  ForceResolutionFrame=World  EnableForceX=on  EnableForceY=on  EnableForceZ=on  EnableForce=off  TorqueResolutionFrame=AttachedFrame  EnableTorqueX=off  EnableTorqueY=off  EnableTorqueZ=off  EnableTorque=off
  Mux : Mux  Inputs=3
  Mux1 : Mux  Inputs=3
  Mux2 : Mux  Inputs=3
  PS-Simulink Converter : nesl_utility/PS-Simulink Converter  PhysicalDomain=network_engine_domain  SubClassName=ps_output  LeftPortType=input  RightPortType=output  PseudoPeriodic=off  Frequencies=[]  VectorFormat=1-D array  Unit=m  AffineConversion=off
      settings: SourceProductBaseCode=PW,SS
  PS-Simulink Converter1 : nesl_utility/PS-Simulink Converter  PhysicalDomain=network_engine_domain  SubClassName=ps_output  LeftPortType=input  RightPortType=output  PseudoPeriodic=off  Frequencies=[]  VectorFormat=1-D array  Unit=m  AffineConversion=off
      settings: SourceProductBaseCode=PW,SS
  PS-Simulink Converter2 : nesl_utility/PS-Simulink Converter  PhysicalDomain=network_engine_domain  SubClassName=ps_output  LeftPortType=input  RightPortType=output  PseudoPeriodic=off  Frequencies=[]  VectorFormat=1-D array  Unit=m  AffineConversion=off
      settings: SourceProductBaseCode=PW,SS
  PS-Simulink Converter3 : nesl_utility/PS-Simulink Converter  PhysicalDomain=network_engine_domain  SubClassName=ps_output  LeftPortType=input  RightPortType=output  PseudoPeriodic=off  Frequencies=[]  VectorFormat=1-D array  Unit=m/s  AffineConversion=off
      settings: SourceProductBaseCode=PW,SS
  PS-Simulink Converter4 : nesl_utility/PS-Simulink Converter  PhysicalDomain=network_engine_domain  SubClassName=ps_output  LeftPortType=input  RightPortType=output  PseudoPeriodic=off  Frequencies=[]  VectorFormat=1-D array  Unit=m/s  AffineConversion=off
      settings: SourceProductBaseCode=PW,SS
  PS-Simulink Converter5 : nesl_utility/PS-Simulink Converter  PhysicalDomain=network_engine_domain  SubClassName=ps_output  LeftPortType=input  RightPortType=output  PseudoPeriodic=off  Frequencies=[]  VectorFormat=1-D array  Unit=m/s  AffineConversion=off
      settings: SourceProductBaseCode=PW,SS
  Simulink-PS Converter : nesl_utility/Simulink-PS Converter  PhysicalDomain=network_engine_domain  SubClassName=ps_input  LeftPortType=input  RightPortType=output  PseudoPeriodic=off  Frequencies=[]  NoiseDistribution=none  NoiseParameters=[]  Unit=N  AffineConversion=off  FilteringAndDerivatives=provide  SimscapeFilterOrder=1  InputFilterTimeConstant=0.001  UdotUserProvided=0
      settings: SourceProductBaseCode=PW,SS
  Simulink-PS Converter1 : nesl_utility/Simulink-PS Converter  PhysicalDomain=network_engine_domain  SubClassName=ps_input  LeftPortType=input  RightPortType=output  PseudoPeriodic=off  Frequencies=[]  NoiseDistribution=none  NoiseParameters=[]  Unit=N  AffineConversion=off  FilteringAndDerivatives=provide  SimscapeFilterOrder=1  InputFilterTimeConstant=0.001  UdotUserProvided=0
      settings: SourceProductBaseCode=PW,SS
  Simulink-PS Converter2 : nesl_utility/Simulink-PS Converter  PhysicalDomain=network_engine_domain  SubClassName=ps_input  LeftPortType=input  RightPortType=output  PseudoPeriodic=off  Frequencies=[]  NoiseDistribution=none  NoiseParameters=[]  Unit=N  AffineConversion=off  FilteringAndDerivatives=provide  SimscapeFilterOrder=1  InputFilterTimeConstant=0.001  UdotUserProvided=0
      settings: SourceProductBaseCode=PW,SS
  Sum : Sum  Inputs=|+-
  Sum1 : Sum
  Terminator : Terminator
  Transform Sensor : sm_lib/Frames and Transforms/Transform Sensor  MeasurementFrame=World  SenseAngle=off  SenseAxis=off  SenseAngle1=off  SenseAngle2=off  SenseAngle3=off  SenseQ=off  SenseR=off  SenseOmegaX=off  SenseOmegaY=off  SenseOmegaZ=off  SenseOmega1=off  SenseOmega2=off  SenseOmega3=off  SenseQDot=off  SenseRDot=off  SenseAlphaX=off  SenseAlphaY=off  SenseAlphaZ=off  SenseAlpha1=off  SenseAlpha2=off  SenseAlpha3=off  SenseQDDot=off  SenseRDDot=off  SenseX=on  SenseY=on  SenseZ=on  SenseRad=off  SenseAzim=off  SenseDist=off  SenseInc=off  SenseXDot=on  SenseYDot=on  SenseZDot=on  SenseRadDot=off  SenseAzimDot=off  SenseDistDot=off  SenseIncDot=off  SenseXDDot=off  SenseYDDot=off  SenseZDDot=off  SenseRadDDot=off  SenseAzimDDot=off  SenseDistDDot=off  SenseIncDDot=off
  contact? : simulink/Logic and Bit Operations/Compare To Zero  relop=<=  OutDataTypeStr=boolean
  z : Selector  InputPortWidth=3  IndexOptions=Index vector (dialog)  Indices=3  OutputSizes=1
  F : PMIOPort  Side=Left
  WorldFrame : PMIOPort  Port=2  Side=Left
  RBallCnt : Outport
  GRF [N N N] : Outport  Port=2
  GRFt [N N N] : Outport  Port=3
  GRFn [N N N] : Outport  Port=4
  wires:
  contact?/1 -> 3D Contact/Enable, RBallCnt/1  "cnt"
  Mux2/1 -> 3D Contact/4(vVec [m/s m/s m/s])
  3D Contact/1(FnVec [N N N]) -> Sum1/1, GRFn [N N N]/1
  3D Contact/2(FtVec [N N N]) -> Sum1/2, GRFt [N N N]/1
  Sum1/1 -> GRF [N N N]/1, Demux1/1
  Sum/1 -> contact?/1
  z/1 -> Sum/1
  Ground/1 -> Mux/3, Sum/2  "EnvHeight"
  Constant1/1 -> 3D Contact/2(nVec [m m m])  "Normal Vector nVec"
  Mux1/1 -> 3D Contact/3(pVec [m m m]), z/1, Demux/1  "Reference Point RefPt"
  Demux/1 -> Mux/1
  Mux/1 -> 3D Contact/1(RefPt [m m m])
  Demux1/1 -> Simulink-PS Converter/1
  Demux1/2 -> Simulink-PS Converter1/1
  Demux1/3 -> Simulink-PS Converter2/1
  PS-Simulink Converter1/1 -> Mux1/2
  PS-Simulink Converter/1 -> Mux1/1
  PS-Simulink Converter2/1 -> Mux1/3
  PS-Simulink Converter3/1 -> Mux2/1
  PS-Simulink Converter4/1 -> Mux2/2
  PS-Simulink Converter5/1 -> Mux2/3
  Demux/3 -> Terminator/1
  Demux/2 -> Mux/2
  connections:
  Transform Sensor/RConn1 -- External Force and Torque/RConn1 -- F/RConn1
  Simulink-PS Converter/RConn1 -- External Force and Torque/LConn1
  Simulink-PS Converter1/RConn1 -- External Force and Torque/LConn2
  Simulink-PS Converter2/RConn1 -- External Force and Torque/LConn3
  WorldFrame/RConn1 -- Transform Sensor/LConn1
  PS-Simulink Converter/LConn1 -- Transform Sensor/RConn2
  PS-Simulink Converter1/LConn1 -- Transform Sensor/RConn3
  PS-Simulink Converter2/LConn1 -- Transform Sensor/RConn4
  PS-Simulink Converter3/LConn1 -- Transform Sensor/RConn5
  PS-Simulink Converter4/LConn1 -- Transform Sensor/RConn6
  PS-Simulink Converter5/LConn1 -- Transform Sensor/RConn7

== system torque_version/Bipedal Model with Torque Control/Right Ball C2 ==
  note: 3D Ground Interaction Model
  Ground : Inport
  3D Contact : Subsystem
  Constant1 : Constant  Value=[0 0 1]
  Demux : Demux  Outputs=3
  Demux1 : Demux  Outputs=3
  External Force and Torque : sm_lib/Forces and Torques/External Force and Torque  ForceResolutionFrame=World  EnableForceX=on  EnableForceY=on  EnableForceZ=on  EnableForce=off  TorqueResolutionFrame=AttachedFrame  EnableTorqueX=off  EnableTorqueY=off  EnableTorqueZ=off  EnableTorque=off
  Mux : Mux  Inputs=3
  Mux1 : Mux  Inputs=3
  Mux2 : Mux  Inputs=3
  PS-Simulink Converter : nesl_utility/PS-Simulink Converter  PhysicalDomain=network_engine_domain  SubClassName=ps_output  LeftPortType=input  RightPortType=output  PseudoPeriodic=off  Frequencies=[]  VectorFormat=1-D array  Unit=m  AffineConversion=off
      settings: SourceProductBaseCode=PW,SS
  PS-Simulink Converter1 : nesl_utility/PS-Simulink Converter  PhysicalDomain=network_engine_domain  SubClassName=ps_output  LeftPortType=input  RightPortType=output  PseudoPeriodic=off  Frequencies=[]  VectorFormat=1-D array  Unit=m  AffineConversion=off
      settings: SourceProductBaseCode=PW,SS
  PS-Simulink Converter2 : nesl_utility/PS-Simulink Converter  PhysicalDomain=network_engine_domain  SubClassName=ps_output  LeftPortType=input  RightPortType=output  PseudoPeriodic=off  Frequencies=[]  VectorFormat=1-D array  Unit=m  AffineConversion=off
      settings: SourceProductBaseCode=PW,SS
  PS-Simulink Converter3 : nesl_utility/PS-Simulink Converter  PhysicalDomain=network_engine_domain  SubClassName=ps_output  LeftPortType=input  RightPortType=output  PseudoPeriodic=off  Frequencies=[]  VectorFormat=1-D array  Unit=m/s  AffineConversion=off
      settings: SourceProductBaseCode=PW,SS
  PS-Simulink Converter4 : nesl_utility/PS-Simulink Converter  PhysicalDomain=network_engine_domain  SubClassName=ps_output  LeftPortType=input  RightPortType=output  PseudoPeriodic=off  Frequencies=[]  VectorFormat=1-D array  Unit=m/s  AffineConversion=off
      settings: SourceProductBaseCode=PW,SS
  PS-Simulink Converter5 : nesl_utility/PS-Simulink Converter  PhysicalDomain=network_engine_domain  SubClassName=ps_output  LeftPortType=input  RightPortType=output  PseudoPeriodic=off  Frequencies=[]  VectorFormat=1-D array  Unit=m/s  AffineConversion=off
      settings: SourceProductBaseCode=PW,SS
  Simulink-PS Converter : nesl_utility/Simulink-PS Converter  PhysicalDomain=network_engine_domain  SubClassName=ps_input  LeftPortType=input  RightPortType=output  PseudoPeriodic=off  Frequencies=[]  NoiseDistribution=none  NoiseParameters=[]  Unit=N  AffineConversion=off  FilteringAndDerivatives=provide  SimscapeFilterOrder=1  InputFilterTimeConstant=0.001  UdotUserProvided=0
      settings: SourceProductBaseCode=PW,SS
  Simulink-PS Converter1 : nesl_utility/Simulink-PS Converter  PhysicalDomain=network_engine_domain  SubClassName=ps_input  LeftPortType=input  RightPortType=output  PseudoPeriodic=off  Frequencies=[]  NoiseDistribution=none  NoiseParameters=[]  Unit=N  AffineConversion=off  FilteringAndDerivatives=provide  SimscapeFilterOrder=1  InputFilterTimeConstant=0.001  UdotUserProvided=0
      settings: SourceProductBaseCode=PW,SS
  Simulink-PS Converter2 : nesl_utility/Simulink-PS Converter  PhysicalDomain=network_engine_domain  SubClassName=ps_input  LeftPortType=input  RightPortType=output  PseudoPeriodic=off  Frequencies=[]  NoiseDistribution=none  NoiseParameters=[]  Unit=N  AffineConversion=off  FilteringAndDerivatives=provide  SimscapeFilterOrder=1  InputFilterTimeConstant=0.001  UdotUserProvided=0
      settings: SourceProductBaseCode=PW,SS
  Sum : Sum  Inputs=|+-
  Sum1 : Sum
  Terminator : Terminator
  Transform Sensor : sm_lib/Frames and Transforms/Transform Sensor  MeasurementFrame=World  SenseAngle=off  SenseAxis=off  SenseAngle1=off  SenseAngle2=off  SenseAngle3=off  SenseQ=off  SenseR=off  SenseOmegaX=off  SenseOmegaY=off  SenseOmegaZ=off  SenseOmega1=off  SenseOmega2=off  SenseOmega3=off  SenseQDot=off  SenseRDot=off  SenseAlphaX=off  SenseAlphaY=off  SenseAlphaZ=off  SenseAlpha1=off  SenseAlpha2=off  SenseAlpha3=off  SenseQDDot=off  SenseRDDot=off  SenseX=on  SenseY=on  SenseZ=on  SenseRad=off  SenseAzim=off  SenseDist=off  SenseInc=off  SenseXDot=on  SenseYDot=on  SenseZDot=on  SenseRadDot=off  SenseAzimDot=off  SenseDistDot=off  SenseIncDot=off  SenseXDDot=off  SenseYDDot=off  SenseZDDot=off  SenseRadDDot=off  SenseAzimDDot=off  SenseDistDDot=off  SenseIncDDot=off
  contact? : simulink/Logic and Bit Operations/Compare To Zero  relop=<=  OutDataTypeStr=boolean
  z : Selector  InputPortWidth=3  IndexOptions=Index vector (dialog)  Indices=3  OutputSizes=1
  F : PMIOPort  Side=Left
  WorldFrame : PMIOPort  Port=2  Side=Left
  RBallCnt : Outport
  GRF [N N N] : Outport  Port=2
  GRFt [N N N] : Outport  Port=3
  GRFn [N N N] : Outport  Port=4
  wires:
  Demux/2 -> Mux/2
  Demux/3 -> Terminator/1
  PS-Simulink Converter5/1 -> Mux2/3
  PS-Simulink Converter4/1 -> Mux2/2
  PS-Simulink Converter3/1 -> Mux2/1
  PS-Simulink Converter2/1 -> Mux1/3
  PS-Simulink Converter/1 -> Mux1/1
  PS-Simulink Converter1/1 -> Mux1/2
  Demux1/3 -> Simulink-PS Converter2/1
  Demux1/2 -> Simulink-PS Converter1/1
  Demux1/1 -> Simulink-PS Converter/1
  Mux/1 -> 3D Contact/1(RefPt [m m m])
  Demux/1 -> Mux/1
  Mux1/1 -> Demux/1, z/1, 3D Contact/3(pVec [m m m])  "Reference Point RefPt"
  Constant1/1 -> 3D Contact/2(nVec [m m m])  "Normal Vector nVec"
  Ground/1 -> Sum/2, Mux/3  "EnvHeight"
  z/1 -> Sum/1
  Sum/1 -> contact?/1
  Sum1/1 -> Demux1/1, GRF [N N N]/1
  3D Contact/2(FtVec [N N N]) -> GRFt [N N N]/1, Sum1/2
  3D Contact/1(FnVec [N N N]) -> GRFn [N N N]/1, Sum1/1
  Mux2/1 -> 3D Contact/4(vVec [m/s m/s m/s])
  contact?/1 -> RBallCnt/1, 3D Contact/Enable  "cnt"
  connections:
  PS-Simulink Converter5/LConn1 -- Transform Sensor/RConn7
  PS-Simulink Converter4/LConn1 -- Transform Sensor/RConn6
  PS-Simulink Converter3/LConn1 -- Transform Sensor/RConn5
  PS-Simulink Converter2/LConn1 -- Transform Sensor/RConn4
  PS-Simulink Converter1/LConn1 -- Transform Sensor/RConn3
  PS-Simulink Converter/LConn1 -- Transform Sensor/RConn2
  WorldFrame/RConn1 -- Transform Sensor/LConn1
  Simulink-PS Converter2/RConn1 -- External Force and Torque/LConn3
  Simulink-PS Converter1/RConn1 -- External Force and Torque/LConn2
  Simulink-PS Converter/RConn1 -- External Force and Torque/LConn1
  F/RConn1 -- External Force and Torque/RConn1 -- Transform Sensor/RConn1
